simulink model "PV_inv_vtg_ctrl"  (R2019a)
settings: Solver=VariableStepAuto  StartTime=0.0  StopTime=5  RelTol=1e-3
values from neighbouring files (symbols this model uses):
  Cfmax = (0.05*P)/(2*pi*f*U^2)    (= 5.51090523171e-06)    [PV_inv_vtg_ctrl_parm.m]
  Lf = ((0.1*U^2)/(2*pi*f*Pmin))    (= 0.00612852634199)    [PV_MPPT_grid.m]    (also in PV_inv_vtg_ctrl_parm.m = 0.00919278951299)
  RLf = Lf*25    (= 0.15321315855)    [PV_MPPT_grid.m]    (also in PV_inv_vtg_ctrl_parm.m = 0.919278951299)
  Tss = 10e-6    (= 1e-05)    [PV_MPPT_grid.m]    (also in PV_inv_vtg_ctrl_parm.m = 5e-06)
libraries: powerlib x10, powerlib_meascontrol x4, dspsrcs4 x3, simulink x1, re_lib x1
settings Model: Creator=nitbh  LastModifiedBy=nitbh

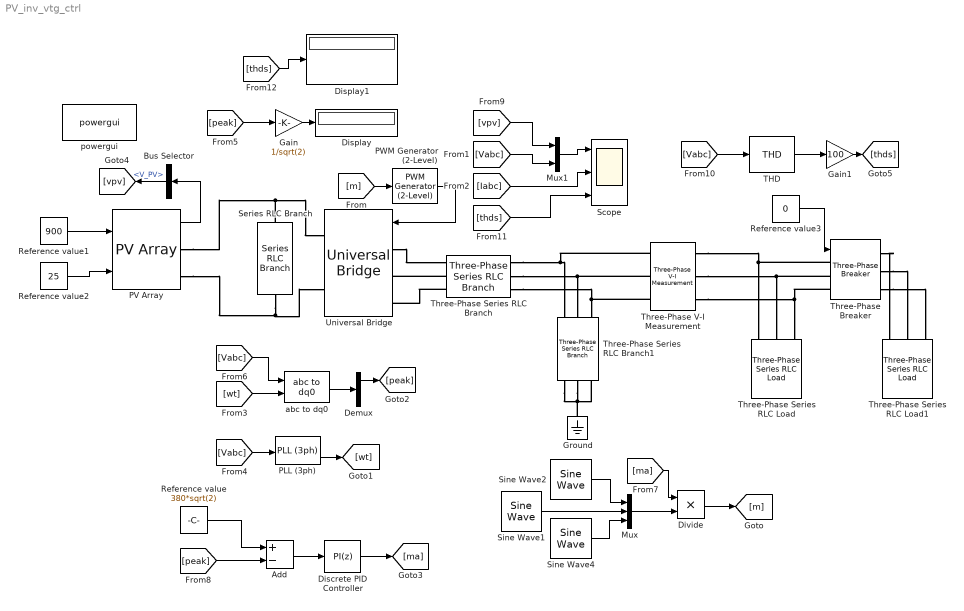
== system PV_inv_vtg_ctrl ==
  Add : Sum  Inputs=+-
  Bus Selector : BusSelector  OutputSignals=V_PV
  Demux : Demux  Outputs=3
  Discrete PID Controller : simulink/Continuous/PID Controller  Controller=PI  Form=Parallel  TimeDomain=Discrete-time  SampleTime=Tss*100  IntegratorMethod=Forward Euler  FilterMethod=Forward Euler  ControllerParametersSource=internal  P=0.001  I=0.6  D=0  UseFilter=on  N=100  TunerSelectOption=Transfer Function Based (PID Tuner App)  InitialConditionSource=internal  InitialConditionForIntegrator=0  InitialConditionForFilter=0  DifferentiatorICPrevScaledInput=0  ExternalReset=none  TrackingMode=off  Kt=1  LimitOutput=on  UpperSaturationLimit=0.95  LowerSaturationLimit=0.3  LinearizeAsGain=off  AntiWindupMode=none  Kb=1  POutMin=[]  POutMax=[]  IOutMin=[]  IOutMax=[]  DOutMin=[]  DOutMax=[]  NOutMin=[]  NOutMax=[]  SumOutMin=[]  SumOutMax=[]  SaturationOutMin=[]  SaturationOutMax=[]  PParamMin=[]  PParamMax=[]  IParamMin=[]  IParamMax=[]  DParamMin=[]  DParamMax=[]  NParamMin=[]  NParamMax=[]  KbParamMin=[]  KbParamMax=[]  KtParamMin=[]  KtParamMax=[]  KbOutMin=[]  KbOutMax=[]  KtOutMin=[]  KtOutMax=[]  IntegratorOutMin=[]  IntegratorOutMax=[]  FilterOutMin=[]  FilterOutMax=[]  SumI1OutMin=[]  SumI1OutMax=[]  SumI2OutMin=[]  SumI2OutMax=[]  SumI3OutMin=[]  SumI3OutMax=[]  SumI4OutMin=[]  SumI4OutMax=[]  SumDOutMin=[]  SumDOutMax=[]  DifferentiatorOutMin=[]  DifferentiatorOutMax=[]  FilterDiffOutCoefMin=[]  FilterDiffOutCoefMax=[]  ReciprocalOutMin=[]  ReciprocalOutMax=[]  SumDenOutMin=[]  SumDenOutMax=[]  SumNumOutMin=[]  SumNumOutMax=[]  DivideOutMin=[]  DivideOutMax=[]  IntegratorContinuousStateAttributes=''  IntegratorStateMustResolveToSignalObject=off  IntegratorRTWStateStorageClass=Auto  FilterContinuousStateAttributes=''  FilterStateMustResolveToSignalObject=off  FilterRTWStateStorageClass=Auto  ParallelPVariant=InternalParameters  IdealPVariant=Disabled  IVariant=InternalParameters  DVariant=Disabled  IntegratorVariant=Discrete  SatVariant=Enabled  AWVariant=Passthrough  PCopyVariant=Disabled  TRVariant=Disabled  FdbkBlocksVariant=Forward  IdealPFdbkVariant=Disabled  SatFdbkVariant=Disabled  DerivativeFilterVariant=Disabled  NVariant=Disabled  NCopyVariant=Disabled_SignalSpec  FilterICVariant=Disabled  IntegratorICVariant=InternalICs  ExternalResetVariant=Disabled  TRSumVariant=Passthrough  SumFdbkVariant=Disabled  SumVariant=Sum_PI
  Display : Display
  Display1 : Display
  Divide : Product  Inputs=**
  Gain : Gain  Gain=1/sqrt(2)
  Gain1 : Gain  Gain=100
  Ground : powerlib/Elements/Ground  LConnTagsString=a
      settings: SourceProductName=Simscape Electrical
  Mux : Mux  Inputs=3
  Mux1 : Mux  Inputs=2
  PLL (3ph) : powerlib_meascontrol/PLL/PLL (3ph)  Fmin=45  Par_Init=[0, 50]  ParK=[180, 3200, 1]  TcD=1e-4  MaxRateChangeFreq=12  FilterCutOffFreq=25  Ts=Tss  AGC=on
      settings: SourceProductName=Simscape Electrical
  PV Array : re_lib/Solar/PV Array  Npar=2  Nser=28  PlotType=array @ 1000 W/m2 & specified temperatures  S_vec="[ 1000  500  100 ]"  Temp_C_vec="[ 45 25  ]"  ModuleName=1Soltech 1STH-215-P  PlotWhenSelected=off  Pm=213.15  Ncell=60  Voc=36.3  Isc=7.84  Vm=29  Im=7.35  beta_Voc_pc=-0.36099  alpha_Isc_pc=0.102  beta_Voc=-0.13104  alpha_Isc=0.007997  IL=7.8649  I0=2.9259e-10  nI=0.98117  Rsh=313.3991  Rs=0.39383  BAL=on  Tc=1e-6  Tfilter=5e-5
      settings: SourceProductName=Simscape Electrical
  PWM Generator (2-Level) : powerlib_meascontrol/Pulse & Signal Generators/PWM Generator (2-Level)  ModulatorType=Three-phase bridge (6 pulses)  ModulatorMode=Unsynchronized  Fc=fsw  Pc=90  nF=27  MinMax="[ -1  1 ]"  SamplingTechnique=Natural  ModulatingSignals=off  m=0.8  Freq=60  Phase=0  Ts=Tss  ShowCarrierOutport=off
  Reference value : Constant  Value=380*sqrt(2)
  Reference value1 : Constant  Value=900
  Reference value2 : Constant  Value=25
  Reference value3 : Constant  Value=0
  Scope : Scope  NumInputPorts=3
  Series RLC Branch : powerlib/Elements/Series RLC Branch  LConnTagsString=__new0  RConnTagsString=__new0  BranchType=RC  Resistance=1  Inductance=1e-3  SetiL0=off  InitialCurrent=0  Capacitance=1000e-6  Setx0=on  InitialVoltage=1000  Measurements=None
      settings: SourceProductName=Simscape Electrical
  Sine Wave1 : dspsrcs4/Sine Wave  Amplitude=1  Frequency=50  Phase=-2*pi/3  SampleMode=Discrete  OutComplex=Real  CompMethod=Trigonometric fcn  TableSize=Speed  SampleTime=Tss  SamplesPerFrame=1  ResetState=Restart at time zero  OutputFrames=off  dataType=double  wordLen=16  udDataType=sfix(16)  fracBitsMode=Best precision  numFracBits=15  OutDataTypeStr=double  LastOutDataTypeStr=double
  Sine Wave2 : dspsrcs4/Sine Wave  Amplitude=1  Frequency=50  Phase=0  SampleMode=Discrete  OutComplex=Real  CompMethod=Trigonometric fcn  TableSize=Speed  SampleTime=Tss  SamplesPerFrame=1  ResetState=Restart at time zero  OutputFrames=off  dataType=double  wordLen=16  udDataType=sfix(16)  fracBitsMode=Best precision  numFracBits=15  OutDataTypeStr=double  LastOutDataTypeStr=double
  Sine Wave4 : dspsrcs4/Sine Wave  Amplitude=1  Frequency=50  Phase=2*pi/3  SampleMode=Discrete  OutComplex=Real  CompMethod=Trigonometric fcn  TableSize=Speed  SampleTime=Tss  SamplesPerFrame=1  ResetState=Restart at time zero  OutputFrames=off  dataType=double  wordLen=16  udDataType=sfix(16)  fracBitsMode=Best precision  numFracBits=15  OutDataTypeStr=double  LastOutDataTypeStr=double
  THD : powerlib_meascontrol/Measurements/THD  Freq=50  Ts=Tss
      settings: SourceProductName=Simscape Electrical
  Three-Phase Series RLC Branch : powerlib/Elements/Three-Phase Series RLC Branch  LConnTagsString=A|B|C  RConnTagsString=A|B|C  BranchType=RL  Resistance=RLf  Inductance=Lf  Capacitance=1e-6  Measurements=None
      settings: SourceProductName=Simscape Electrical
  Three-Phase Series RLC Branch1 : powerlib/Elements/Three-Phase Series RLC Branch  LConnTagsString=A|B|C  RConnTagsString=A|B|C  BranchType=RC  Resistance=1e-6  Inductance=Lf  Capacitance=Cfmax  Measurements=None
      settings: SourceProductName=Simscape Electrical
  Three-Phase Series RLC Load : powerlib/Elements/Three-Phase Series RLC Load  LConnTagsString=A|B|C  Configuration=Y (grounded)  NominalVoltage=380  Vabc=[1e3 1e3 1e3]  Vabcp=[1e3 1e3 1e3]  NominalFrequency=50  UnbalancedPower=off  ActivePower=5e3  InductivePower=0  CapacitivePower=0  Pabc=[10e3 9e3 11e3]  QLabc=[100 90 110]  QCabc=[100 90 110]  Pabcp=[10e3 9e3 11e3]  QLabcp=[100 90 110]  QCabcp=[100 90 110]  Measurements=None  LoadType=constant Z
      settings: SourceProductName=Simscape Electrical
  Three-Phase Series RLC Load1 : powerlib/Elements/Three-Phase Series RLC Load  LConnTagsString=A|B|C  Configuration=Y (grounded)  NominalVoltage=380  Vabc=[1e3 1e3 1e3]  Vabcp=[1e3 1e3 1e3]  NominalFrequency=50  UnbalancedPower=off  ActivePower=5e3  InductivePower=0  CapacitivePower=0  Pabc=[10e3 9e3 11e3]  QLabc=[100 90 110]  QCabc=[100 90 110]  Pabcp=[10e3 9e3 11e3]  QLabcp=[100 90 110]  QCabcp=[100 90 110]  Measurements=None  LoadType=constant Z
      settings: SourceProductName=Simscape Electrical
  Three-Phase V-I Measurement : powerlib/Measurements/Three-Phase V-I Measurement  VoltageMeasurement=phase-to-phase  SetLabelV=on  LabelV=Vabc  Vpu=off  VpuLL=off  CurrentMeasurement=yes  SetLabelI=on  LabelI=Iabc  Ipu=off  Pbase=100e6  Vbase=500e3  OutputType=Complex  PhasorSimulation=off  PSBequivalent=0
      settings: SourceProductName=Simscape Electrical
  Three-Phase Breaker : powerlib/Elements/Three-Phase Breaker  InitialState=open  SwitchA=on  SwitchB=on  SwitchC=on  SwitchTimes="[1/60  5/60]"  External=on  BreakerResistance=0.01  SnubberResistance=1e6  SnubberCapacitance=inf  Measurements=None
      settings: SourceProductName=Simscape Electrical
  Universal Bridge : powerlib/Power Electronics/Universal Bridge  Arms=3  SnubberResistance=1e5  SnubberCapacitance=inf  Device=IGBT / Diodes  Ron=1e-3  Lon=0  ForwardVoltages="[  0  0  ]"  ForwardVoltage=0  GTOparameters=[ 10e-6 , 20e-6 ]  IGBTparameters=[ 1e-6 , 2e-6 ]  Measurements=None  Measurements_2=None  converterType=Rectifier
      settings: SourceProductName=Simscape Electrical
  abc to dq0 : powerlib_meascontrol/Transformations/abc to dq0  Alignment=90 degrees behind phase A axis
      settings: SourceProductName=Simscape Electrical
  powergui : powerlib/powergui  Priority=1  SimulationMode=Discrete  SampleTime=Tss  frequency=60  Iterations=50  frequencyindice=0  Pbase=100e6  ErrMax=1e-4  UnitsV=kV  UnitsW=MW  buscounter=0  FunctionMessages=off  echomessages=off  EnableUseOfTLC=off  CurrentSourceSwitches=off  DisableSnubberDevices=off  DisableRonSwitches=off  DisableVfSwitches=off  DisplayEquations=off  AutomaticDiscreteSolvers=off  SolverType=Tustin/Backward Euler (TBE)  Interpol=off  ExternalGateDelay=off  methode=off  Ts=100  x0status=blocks  SPID=on  SwTol=0  HookPort=off  NonlinearTolerance=0  nMaxIteration=15  ContinueOnMaxIteration=off  RestoreLinks=warning  ResistiveCurrentMeasurement=off  Frange=[0:2:500]  Ylog=off  Xlog=on  ShowGrid=off  save=off  variable=ZData  structure=0  ZoomFFT=off  StartTime=0.0  cycles=1  DisplayStyle=1  fundamental=60  FreqAxis=off  MaxFrequency=1000  frequencyindicesteady=1  RmsSteady=1  display=off
      settings: SourceProductName=Simscape Electrical
  wires:
  [m] -> PWM Generator (2-Level)/1
  PWM Generator (2-Level)/1 -> Universal Bridge/1
  Sine Wave2/1 -> Mux/1
  Sine Wave1/1 -> Mux/2
  Sine Wave4/1 -> Mux/3
  [Iabc] -> Scope/2
  [wt] -> abc to dq0/2
  [Vabc] -> abc to dq0/1
  abc to dq0/1 -> Demux/1
  PLL (3ph)/2 -> [wt]
  [Vabc] -> PLL (3ph)/1
  Demux/1 -> [peak]
  [peak] -> Gain/1
  Gain/1 -> Display/1
  Discrete PID Controller/1 -> [ma]
  Add/1 -> Discrete PID Controller/1
  Mux/1 -> Divide/2
  Divide/1 -> [m]
  [ma] -> Divide/1
  [peak] -> Add/2
  Reference value/1 -> Add/1
  PV Array/1 -> Bus Selector/1
  Bus Selector/1 -> [vpv]  "<V_PV>"
  Mux1/1 -> Scope/1
  [Vabc] -> Mux1/2
  [vpv] -> Mux1/1
  Reference value1/1 -> PV Array/1
  Reference value2/1 -> PV Array/2
  Reference value3/1 -> Three-Phase Breaker/1
  [Vabc] -> THD/1
  THD/1 -> Gain1/1
  Gain1/1 -> [thds]
  [thds] -> Scope/3
  [thds] -> Display1/1
  connections:
  Three-Phase Series RLC Branch/LConn2 -- Universal Bridge/LConn2
  Universal Bridge/LConn1 -- Three-Phase Series RLC Branch/LConn1
  Three-Phase Series RLC Branch/LConn3 -- Universal Bridge/LConn3
  Three-Phase Series RLC Branch/RConn3 -- Three-Phase V-I Measurement/LConn3 -- Three-Phase Series RLC Branch1/LConn3
  Three-Phase Series RLC Branch/RConn2 -- Three-Phase V-I Measurement/LConn2 -- Three-Phase Series RLC Branch1/LConn2
  Three-Phase Series RLC Branch/RConn1 -- Three-Phase V-I Measurement/LConn1 -- Three-Phase Series RLC Branch1/LConn1
  Three-Phase Series RLC Branch1/RConn1 -- Ground/LConn1 -- Three-Phase Series RLC Branch1/RConn2 -- Three-Phase Series RLC Branch1/RConn3
  Three-Phase V-I Measurement/RConn3 -- Three-Phase Breaker/LConn3 -- Three-Phase Series RLC Load/LConn3
  Three-Phase V-I Measurement/RConn2 -- Three-Phase Breaker/LConn2 -- Three-Phase Series RLC Load/LConn2
  Three-Phase V-I Measurement/RConn1 -- Three-Phase Breaker/LConn1 -- Three-Phase Series RLC Load/LConn1
  Series RLC Branch/LConn1 -- PV Array/RConn1 -- Universal Bridge/RConn1
  Series RLC Branch/RConn1 -- PV Array/RConn2 -- Universal Bridge/RConn2
  Three-Phase Breaker/RConn3 -- Three-Phase Series RLC Load1/LConn3
  Three-Phase Breaker/RConn2 -- Three-Phase Series RLC Load1/LConn2
  Three-Phase Breaker/RConn1 -- Three-Phase Series RLC Load1/LConn1
